simulink model "AdaptivePI_Simulation"  (R2020a)
settings: Solver=ode45  StartTime=0  StopTime=800  MaxStep=0.2  RelTol=1e-3  EnableMultiTasking=on
model workspace (MATLAB code in the model file):
  | %Model constants
  | k0                = 34930800;
  | DeltaER       = 5963.6;
  | DeltaH         = -11.92;
  | UA               = 0.3;
  | FV_plus_UA = 1.3;
  | 
  | %Fixed IC
  | Concentration0 = 1.5;
  | FeedCon0         = 10;
  | FeedTemp0       = 295;
  | 
  | %Derived IC
  | tmpVal = FeedCon0/Concentration0-1;
  | ReactorTemp0 = -DeltaER/log(tmpVal/k0);
  | CoolantTemp0 = (ReactorTemp0*(FV_plus_UA)+tmpVal*Concentration0*DeltaH-FeedTemp0)/UA;
  | 
  | %
  | tStep = 400; % [s] When the step reference change happens
  | Ts = 0.1; % [s] Sample time
  | 
  | % Scaling factors on the signals
  | CAscale = 10;
  | Tcscale = 1/10;
  | 
  | % Moving average filter
  | N = 100;
  | 
  | %Clean up
  | clear tmpVal
libraries: simulink x5
settings Model: OrderedModelArguments=off  Creator=The MathWorks, Inc.  LastModifiedBy=Mirza
settings DataIOCC: InitialState=[311.267; 8.5695]  SaveFormat=Array  SaveOutput=off  SignalLogging=off  DSMLogging=off  SaveTime=off  ReturnWorkspaceOutputs=off  SignalLoggingName=logsOut
settings OptimizationCC: BlockReduction=off  BooleanDataType=off  DefaultParameterBehavior=Inlined  InlineInvariantSignals=on  BufferReuse=off  ExpressionDepthLimit=2147483647  InitFltsAndDblsToZero=on  LifeSpan=inf
settings DebuggingCC: SaveWithParameterizedLinksMsg=none  UnderspecifiedInitializationDetection=Classic  MergeDetectMultiDrivingBlocksExec=none  CheckExecutionContextPreStartOutputMsg=on  CheckExecutionContextRuntimeOutputMsg=on  SignalResolutionControl=TryResolveAllWithWarning  MultiTaskDSMMsg=warning  MultiTaskCondExecSysMsg=none  FcnCallInpInsideContextMsg=warning  AllowSymbolicDim=off  StateNameClashWarn=warning  SFUnexpectedBacktrackingDiag=warning  SFNoUnconditionalDefaultTransitionDiag=warning  SFExecutionAtInitializationDiag=none  ArithmeticOperatorsInVariantConditions=warning
settings HardwareCC: ProdBitPerPointer=32  ProdBitPerSizeT=32  ProdBitPerPtrDiffT=32  ProdLargestAtomicFloat=None  ProdIntDivRoundTo=Undefined  ProdEndianess=Unspecified  ProdWordSize=32  ProdHWDeviceType=32-bit Generic  TargetUnknown=on
settings ModelReferenceCC: PropagateSignalLabelsOutOfModel=off
settings SFSimCC: SimUseLocalCustomCode=off  CustomCodeUndefinedFunction=UseInterfaceOnly
settings RTWCC: RTWUseLocalCustomCode=off
settings CodeAppCC: StateflowObjectComments=on
settings GRTTargetCC: TargetFcnLib=ansi_tfl_tmw.mat  TargetLangStandard=C89/C90 (ANSI)  CombineOutputUpdateFcns=off  GRTInterface=on
settings ConfigComp: CovMetricSettings=dw  CovHtmlReporting=on  CovSaveCumulativeToWorkspaceVar=on  CovSaveSingleToWorkspaceVar=on  CovExternalEMLEnable=off  CovSFcnEnable=off

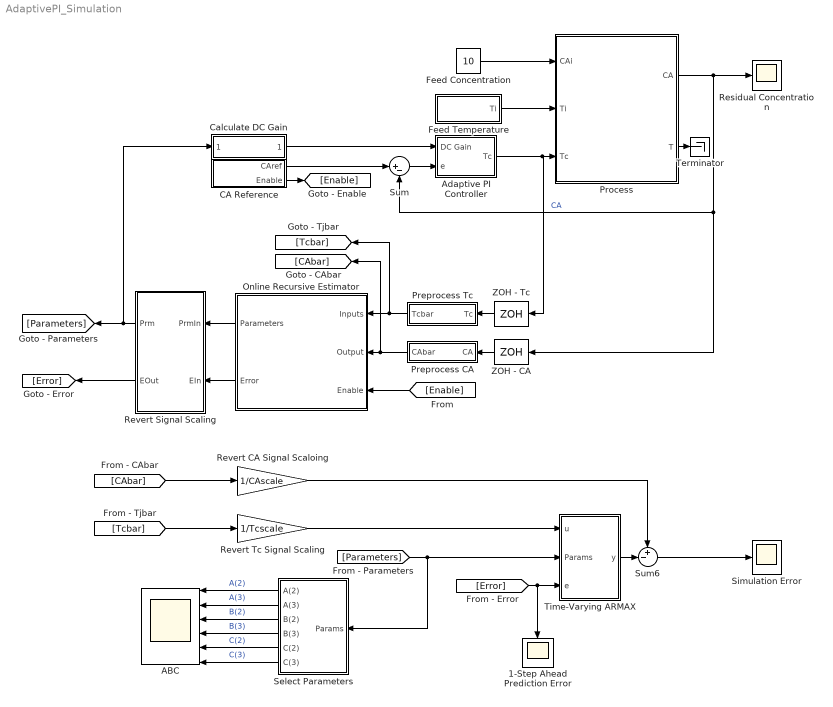
== system AdaptivePI_Simulation ==
  " Revert CA Signal Scaloing" : Gain  Gain=1/CAscale
  1-Step Ahead Prediction Error : Scope
  ABC : Scope  NumInputPorts=6
  Adaptive PI Controller : Subsystem
  CA Reference : Subsystem
  Calculate DC Gain : Subsystem
  Feed Concentration : Constant  Value=10
  Feed Temperature : Subsystem
  Online Recursive Estimator : Subsystem  mask{ModelStructure=ARMAX, A0=2, B0=[2], F0=2, C0=2, D0=2, d=[0], P0=100, History=Infinitna, WindowLength=2000, EstimationMethod=Faktor iscezavanja, Lambda=1 - 5e-3, ProcessNoiseCovariance=0.01, Tolerance=0.0001, AddEnablePort=on, EstimationError=on, ExcitationMeasure=off, SampleTime=0.1}
      mask prompts: ModelStructure "Izbor modela:"; A0 "Broj parametara u A(q) (na):"; B0 "Broj parametara u B(q) (nb):"; F0 "Broj parametara u F(q) (nf):"; C0 "Broj parametara u C(q) (nc):"; D0 "Broj parametara u D(q) (nd):"; d "Kasnjenje ulaza (nk):"; P0 "Matrica kovarijanse parametara:"; History "Historija:"; WindowLength "Sirina prozora:"; EstimationMethod "Metod estimacije:"; Lambda "Faktor iscezavanja:"; ProcessNoiseCovariance "Kovarijansa procesnog suma:"; Tolerance "Toleranca:"; AddEnablePort "Enable port"; EstimationError "Greska estimacije:"; ExcitationMeasure "Mjera pobude:"; SampleTime "Period uzorkovanja:"
      mask TypeOptions ModelStructure: ARX | ARMAX | BJ | OE
      mask Callback ModelStructure:
      | maskStr = get_param(gcb, 'ModelStructure');
      | maskStr1 = get_param(gcb, 'History');
      | maskStr2 = get_param(gcb, 'EstimationMethod');
      | 
      | if strcmp(maskStr, 'ARX') && strcmp(maskStr1, 'Infinitna') && strcmp(maskStr2, 'Faktor iscezavanja') ,
      |     set_param(gcb, 'MaskVisibilities', {'on';'on';'on';'off';'off';'off';'on';'on';'on';'off';'on';'on';'off';'off';'on';'on';'on';'on'}),
      | elseif strcmp(maskStr, 'ARX') && strcmp(maskStr1, 'Infinitna') && strcmp(maskStr2, 'BFGS') ,
      |     set_param(gcb, 'MaskVisibilities', {'on';'on';'on';'off';'off';'off';'on';'on';'on';'on';'on';'off';'off';'on';'on';'on';'on';'on'}),
      | elseif strcmp(maskStr, 'ARX') && strcmp(maskStr1, 'Infinitna') && strcmp(maskStr2, 'Kalmanov filter') ,
      |     set_param(gcb, 'MaskVisibilities', {'on';'on';'on';'off';'off';'off';'on';'on';'on';'off';'on';'off';'on';'off';'on';'on';'on';'on'}),
      | elseif strcmp(maskStr, 'ARX') && strcmp(maskStr1, 'Finitna') && strcmp(maskStr2, 'Faktor iscezavanja') ,
      |     set_param(gcb, 'MaskVisibilities', {'on';'on';'on';'off';'off';'off';'on';'on';'on';'on';'on';'off';'off';'off';'on';'on';'on';'on'}),
      | elseif strcmp(maskStr, 'ARX') && strcmp(maskStr1, 'Finitna') && strcmp(maskStr2, 'BFGS') ,
      |     set_param(gcb, 'MaskVisibilities', {'on';'on';'on';'off';'off';'off';'on';'on';'on';'on';'on';'off';'off';'on';'on';'on';'on';'on'}),
      | elseif strcmp(maskStr, 'ARX') && strcmp(maskStr1, 'Finitna') && strcmp(maskStr2, 'Kalmanov filter') ,
      |     set_param(gcb, 'MaskVisibilities', {'on';'on';'on';'off';'off';'off';'on';'on';'on';'on';'on';'off';'off';'off';'on';'on';'on';'on'}),
      | elseif strcmp(maskStr, 'ARMAX') && strcmp(maskStr1, 'Infinitna') && strcmp(maskStr2, 'Faktor iscezavanja') ,
      |     set_param(gcb, 'MaskVisibilities', {'on';'on';'on';'off';'on';'off';'on';'on';'on';'off';'on';'on';'off';'off';'on';'on';'on';'on'}),
      | elseif strcmp(maskStr, 'ARMAX') && strcmp(maskStr1, 'Infinitna') && strcmp(maskStr2, 'BFGS') ,
      |     set_param(gcb, 'MaskVisibilities', {'on';'on';'on';'off';'on';'off';'on';'on';'on';'on';'on';'off';'off';'on';'on';'on';'on';'on'}),
      | elseif strcmp(maskStr, 'ARMAX') && strcmp(maskStr1, 'Infinitna') && strcmp(maskStr2, 'Kalmanov filter') ,
      |     set_param(gcb, 'MaskVisibilities', {'on';'on';'on';'off';'on';'off';'on';'on';'on';'off';'on';'off';'on';'off';'on';'on';'on';'on'}),
      | elseif strcmp(maskStr, 'ARMAX') && strcmp(maskStr1, 'Finitna') && strcmp(maskStr2, 'Faktor iscezavanja') ,
      |     set_param(gcb, 'MaskVisibilities', {'on';'on';'on';'off';'on';'off';'on';'on';'on';'on';'on';'off';'off';'off';'on';'on';'on';'on'}),
      | elseif strcmp(maskStr, 'ARMAX') && strcmp(maskStr1, 'Finitna') && strcmp(maskStr2, 'BFGS') ,
      |     set_param(gcb, 'MaskVisibilities', {'on';'on';'on';'off';'on';'off';'on';'on';'on';'on';'on';'off';'off';'on';'on';'on';'on';'on'}),
      | elseif strcmp(maskStr, 'ARMAX') && strcmp(maskStr1, 'Finitna') && strcmp(maskStr2, 'Kalmanov filter') ,
      |     set_param(gcb, 'MaskVisibilities', {'on';'on';'on';'off';'on';'off';'on';'on';'on';'on';'on';'off';'off';'off';'on';'on';'on';'on'}),
      | elseif strcmp(maskStr, 'BJ') && strcmp(maskStr1, 'Infinitna') && strcmp(maskStr2, 'Faktor iscezavanja') ,
      |     set_param(gcb, 'MaskVisibilities', {'on';'off';'on';'on';'on';'on';'on';'on';'on';'off';'on';'on';'off';'off';'on';'on';'on';'on'}),
      | elseif strcmp(maskStr, 'BJ') && strcmp(maskStr1, 'Infinitna') && strcmp(maskStr2, 'BFGS') ,
      |     set_param(gcb, 'MaskVisibilities', {'on';'off';'on';'on';'on';'on';'on';'on';'on';'on';'on';'off';'off';'on';'on';'on';'on';'on'}),
      | elseif strcmp(maskStr, 'BJ') && strcmp(maskStr1, 'Infinitna') && strcmp(maskStr2, 'Kalmanov filter') ,
      |     set_param(gcb, 'MaskVisibilities', {'on';'off';'on';'on';'on';'on';'on';'on';'on';'off';'on';'off';'on';'off';'on';'on';'on';'on'}),
      | elseif strcmp(maskStr, 'BJ') && strcmp(maskStr1, 'Finitna') && strcmp(maskStr2, 'Faktor iscezavanja') ,
      |     set_param(gcb, 'MaskVisibilities', {'on';'off';'on';'on';'on';'on';'on';'on';'on';'on';'on';'off';'off';'off';'on';'on';'on';'on'}),
      | elseif strcmp(maskStr, 'BJ') && strcmp(maskStr1, 'Finitna') && strcmp(maskStr2, 'BFGS') ,
      |     set_param(gcb, 'MaskVisibilities', {'on';'off';'on';'on';'on';'on';'on';'on';'on';'on';'on';'off';'off';'on';'on';'on';'on';'on'}),
      | elseif strcmp(maskStr, 'BJ') && strcmp(maskStr1, 'Finitna') && strcmp(maskStr2, 'Kalmanov filter') ,
      |     set_param(gcb, 'MaskVisibilities', {'on';'off';'on';'on';'on';'on';'on';'on';'on';'on';'on';'off';'off';'off';'on';'on';'on';'on'}),
      | elseif strcmp(maskStr, 'OE') && strcmp(maskStr1, 'Infinitna') && strcmp(maskStr2, 'Faktor iscezavanja') ,
      |     set_param(gcb, 'MaskVisibilities', {'on';'off';'on';'on';'off';'off';'on';'on';'on';'off';'on';'on';'off';'off';'on';'on';'on';'on'}),
      | elseif strcmp(maskStr, 'OE') && strcmp(maskStr1, 'Infinitna') && strcmp(maskStr2, 'BFGS') ,
      |     set_param(gcb, 'MaskVisibilities', {'on';'off';'on';'on';'off';'off';'on';'on';'on';'on';'on';'off';'off';'on';'on';'on';'on';'on'}),
      | elseif strcmp(maskStr, 'OE') && strcmp(maskStr1, 'Infinitna') && strcmp(maskStr2, 'Kalmanov filter') ,
      |     set_param(gcb, 'MaskVisibilities', {'on';'off';'on';'on';'off';'off';'on';'on';'on';'off';'on';'off';'on';'off';'on';'on';'on';'on'}),
      | elseif strcmp(maskStr, 'OE') && strcmp(maskStr1, 'Finitna') && strcmp(maskStr2, 'Faktor iscezavanja') ,
      |     set_param(gcb, 'MaskVisibilities', {'on';'off';'on';'on';'off';'off';'on';'on';'on';'on';'on';'off';'off';'off';'on';'on';'on';'on'}),
      | elseif strcmp(maskStr, 'OE') && strcmp(maskStr1, 'Finitna') && strcmp(maskStr2, 'BFGS') ,
      |     set_param(gcb, 'MaskVisibilities', {'on';'off';'on';'on';'off';'off';'on';'on';'on';'on';'on';'off';'off';'on';'on';'on';'on';'on'}),
      | elseif strcmp(maskStr, 'OE') && strcmp(maskStr1, 'Finitna') && strcmp(maskStr2, 'Kalmanov filter') ,
      |     set_param(gcb, 'MaskVisibilities', {'on';'off';'on';'on';'off';'off';'on';'on';'on';'on';'on';'off';'off';'off';'on';'on';'on';'on'}),
      | end
      mask TypeOptions History: Infinitna | Finitna
      mask Callback History:
      | maskStr = get_param(gcb, 'ModelStructure');
      | maskStr1 = get_param(gcb, 'History');
      | maskStr2 = get_param(gcb, 'EstimationMethod');
      | 
      | if strcmp(maskStr, 'ARX') && strcmp(maskStr1, 'Infinitna') && strcmp(maskStr2, 'Faktor iscezavanja') ,
      |     set_param(gcb, 'MaskVisibilities', {'on';'on';'on';'off';'off';'off';'on';'on';'on';'off';'on';'on';'off';'off';'on';'on';'on';'on'}),
      | elseif strcmp(maskStr, 'ARX') && strcmp(maskStr1, 'Infinitna') && strcmp(maskStr2, 'BFGS') ,
      |     set_param(gcb, 'MaskVisibilities', {'on';'on';'on';'off';'off';'off';'on';'on';'on';'on';'on';'off';'off';'on';'on';'on';'on';'on'}),
      | elseif strcmp(maskStr, 'ARX') && strcmp(maskStr1, 'Infinitna') && strcmp(maskStr2, 'Kalmanov filter') ,
      |     set_param(gcb, 'MaskVisibilities', {'on';'on';'on';'off';'off';'off';'on';'on';'on';'off';'on';'off';'on';'off';'on';'on';'on';'on'}),
      | elseif strcmp(maskStr, 'ARX') && strcmp(maskStr1, 'Finitna') && strcmp(maskStr2, 'Faktor iscezavanja') ,
      |     set_param(gcb, 'MaskVisibilities', {'on';'on';'on';'off';'off';'off';'on';'on';'on';'on';'on';'off';'off';'off';'on';'on';'on';'on'}),
      | elseif strcmp(maskStr, 'ARX') && strcmp(maskStr1, 'Finitna') && strcmp(maskStr2, 'BFGS') ,
      |     set_param(gcb, 'MaskVisibilities', {'on';'on';'on';'off';'off';'off';'on';'on';'on';'on';'on';'off';'off';'on';'on';'on';'on';'on'}),
      | elseif strcmp(maskStr, 'ARX') && strcmp(maskStr1, 'Finitna') && strcmp(maskStr2, 'Kalmanov filter') ,
      |     set_param(gcb, 'MaskVisibilities', {'on';'on';'on';'off';'off';'off';'on';'on';'on';'on';'on';'off';'off';'off';'on';'on';'on';'on'}),
      | elseif strcmp(maskStr, 'ARMAX') && strcmp(maskStr1, 'Infinitna') && strcmp(maskStr2, 'Faktor iscezavanja') ,
      |     set_param(gcb, 'MaskVisibilities', {'on';'on';'on';'off';'on';'off';'on';'on';'on';'off';'on';'on';'off';'off';'on';'on';'on';'on'}),
      | elseif strcmp(maskStr, 'ARMAX') && strcmp(maskStr1, 'Infinitna') && strcmp(maskStr2, 'BFGS') ,
      |     set_param(gcb, 'MaskVisibilities', {'on';'on';'on';'off';'on';'off';'on';'on';'on';'on';'on';'off';'off';'on';'on';'on';'on';'on'}),
      | elseif strcmp(maskStr, 'ARMAX') && strcmp(maskStr1, 'Infinitna') && strcmp(maskStr2, 'Kalmanov filter') ,
      |     set_param(gcb, 'MaskVisibilities', {'on';'on';'on';'off';'on';'off';'on';'on';'on';'off';'on';'off';'on';'off';'on';'on';'on';'on'}),
      | elseif strcmp(maskStr, 'ARMAX') && strcmp(maskStr1, 'Finitna') && strcmp(maskStr2, 'Faktor iscezavanja') ,
      |     set_param(gcb, 'MaskVisibilities', {'on';'on';'on';'off';'on';'off';'on';'on';'on';'on';'on';'off';'off';'off';'on';'on';'on';'on'}),
      | elseif strcmp(maskStr, 'ARMAX') && strcmp(maskStr1, 'Finitna') && strcmp(maskStr2, 'BFGS') ,
      |     set_param(gcb, 'MaskVisibilities', {'on';'on';'on';'off';'on';'off';'on';'on';'on';'on';'on';'off';'off';'on';'on';'on';'on';'on'}),
      | elseif strcmp(maskStr, 'ARMAX') && strcmp(maskStr1, 'Finitna') && strcmp(maskStr2, 'Kalmanov filter') ,
      |     set_param(gcb, 'MaskVisibilities', {'on';'on';'on';'off';'on';'off';'on';'on';'on';'on';'on';'off';'off';'off';'on';'on';'on';'on'}),
      | elseif strcmp(maskStr, 'BJ') && strcmp(maskStr1, 'Infinitna') && strcmp(maskStr2, 'Faktor iscezavanja') ,
      |     set_param(gcb, 'MaskVisibilities', {'on';'off';'on';'on';'on';'on';'on';'on';'on';'off';'on';'on';'off';'off';'on';'on';'on';'on'}),
      | elseif strcmp(maskStr, 'BJ') && strcmp(maskStr1, 'Infinitna') && strcmp(maskStr2, 'BFGS') ,
      |     set_param(gcb, 'MaskVisibilities', {'on';'off';'on';'on';'on';'on';'on';'on';'on';'on';'on';'off';'off';'on';'on';'on';'on';'on'}),
      | elseif strcmp(maskStr, 'BJ') && strcmp(maskStr1, 'Infinitna') && strcmp(maskStr2, 'Kalmanov filter') ,
      |     set_param(gcb, 'MaskVisibilities', {'on';'off';'on';'on';'on';'on';'on';'on';'on';'off';'on';'off';'on';'off';'on';'on';'on';'on'}),
      | elseif strcmp(maskStr, 'BJ') && strcmp(maskStr1, 'Finitna') && strcmp(maskStr2, 'Faktor iscezavanja') ,
      |     set_param(gcb, 'MaskVisibilities', {'on';'off';'on';'on';'on';'on';'on';'on';'on';'on';'on';'off';'off';'off';'on';'on';'on';'on'}),
      | elseif strcmp(maskStr, 'BJ') && strcmp(maskStr1, 'Finitna') && strcmp(maskStr2, 'BFGS') ,
      |     set_param(gcb, 'MaskVisibilities', {'on';'off';'on';'on';'on';'on';'on';'on';'on';'on';'on';'off';'off';'on';'on';'on';'on';'on'}),
      | elseif strcmp(maskStr, 'BJ') && strcmp(maskStr1, 'Finitna') && strcmp(maskStr2, 'Kalmanov filter') ,
      |     set_param(gcb, 'MaskVisibilities', {'on';'off';'on';'on';'on';'on';'on';'on';'on';'on';'on';'off';'off';'off';'on';'on';'on';'on'}),
      | elseif strcmp(maskStr, 'OE') && strcmp(maskStr1, 'Infinitna') && strcmp(maskStr2, 'Faktor iscezavanja') ,
      |     set_param(gcb, 'MaskVisibilities', {'on';'off';'on';'on';'off';'off';'on';'on';'on';'off';'on';'on';'off';'off';'on';'on';'on';'on'}),
      | elseif strcmp(maskStr, 'OE') && strcmp(maskStr1, 'Infinitna') && strcmp(maskStr2, 'BFGS') ,
      |     set_param(gcb, 'MaskVisibilities', {'on';'off';'on';'on';'off';'off';'on';'on';'on';'on';'on';'off';'off';'on';'on';'on';'on';'on'}),
      | elseif strcmp(maskStr, 'OE') && strcmp(maskStr1, 'Infinitna') && strcmp(maskStr2, 'Kalmanov filter') ,
      |     set_param(gcb, 'MaskVisibilities', {'on';'off';'on';'on';'off';'off';'on';'on';'on';'off';'on';'off';'on';'off';'on';'on';'on';'on'}),
      | elseif strcmp(maskStr, 'OE') && strcmp(maskStr1, 'Finitna') && strcmp(maskStr2, 'Faktor iscezavanja') ,
      |     set_param(gcb, 'MaskVisibilities', {'on';'off';'on';'on';'off';'off';'on';'on';'on';'on';'on';'off';'off';'off';'on';'on';'on';'on'}),
      | elseif strcmp(maskStr, 'OE') && strcmp(maskStr1, 'Finitna') && strcmp(maskStr2, 'BFGS') ,
      |     set_param(gcb, 'MaskVisibilities', {'on';'off';'on';'on';'off';'off';'on';'on';'on';'on';'on';'off';'off';'on';'on';'on';'on';'on'}),
      | elseif strcmp(maskStr, 'OE') && strcmp(maskStr1, 'Finitna') && strcmp(maskStr2, 'Kalmanov filter') ,
      |     set_param(gcb, 'MaskVisibilities', {'on';'off';'on';'on';'off';'off';'on';'on';'on';'on';'on';'off';'off';'off';'on';'on';'on';'on'}),
      | end
      mask TypeOptions EstimationMethod: Faktor iscezavanja | BFGS | Kalmanov filter
      mask Callback EstimationMethod:
      | maskStr = get_param(gcb, 'ModelStructure');
      | maskStr1 = get_param(gcb, 'History');
      | maskStr2 = get_param(gcb, 'EstimationMethod');
      | 
      | if strcmp(maskStr, 'ARX') && strcmp(maskStr1, 'Infinitna') && strcmp(maskStr2, 'Faktor iscezavanja') ,
      |     set_param(gcb, 'MaskVisibilities', {'on';'on';'on';'off';'off';'off';'on';'on';'on';'off';'on';'on';'off';'off';'on';'on';'on';'on'}),
      | elseif strcmp(maskStr, 'ARX') && strcmp(maskStr1, 'Infinitna') && strcmp(maskStr2, 'BFGS') ,
      |     set_param(gcb, 'MaskVisibilities', {'on';'on';'on';'off';'off';'off';'on';'on';'on';'on';'on';'off';'off';'on';'on';'on';'on';'on'}),
      | elseif strcmp(maskStr, 'ARX') && strcmp(maskStr1, 'Infinitna') && strcmp(maskStr2, 'Kalmanov filter') ,
      |     set_param(gcb, 'MaskVisibilities', {'on';'on';'on';'off';'off';'off';'on';'on';'on';'off';'on';'off';'on';'off';'on';'on';'on';'on'}),
      | elseif strcmp(maskStr, 'ARX') && strcmp(maskStr1, 'Finitna') && strcmp(maskStr2, 'Faktor iscezavanja') ,
      |     set_param(gcb, 'MaskVisibilities', {'on';'on';'on';'off';'off';'off';'on';'on';'on';'on';'on';'off';'off';'off';'on';'on';'on';'on'}),
      | elseif strcmp(maskStr, 'ARX') && strcmp(maskStr1, 'Finitna') && strcmp(maskStr2, 'BFGS') ,
      |     set_param(gcb, 'MaskVisibilities', {'on';'on';'on';'off';'off';'off';'on';'on';'on';'on';'on';'off';'off';'on';'on';'on';'on';'on'}),
      | elseif strcmp(maskStr, 'ARX') && strcmp(maskStr1, 'Finitna') && strcmp(maskStr2, 'Kalmanov filter') ,
      |     set_param(gcb, 'MaskVisibilities', {'on';'on';'on';'off';'off';'off';'on';'on';'on';'on';'on';'off';'off';'off';'on';'on';'on';'on'}),
      | elseif strcmp(maskStr, 'ARMAX') && strcmp(maskStr1, 'Infinitna') && strcmp(maskStr2, 'Faktor iscezavanja') ,
      |     set_param(gcb, 'MaskVisibilities', {'on';'on';'on';'off';'on';'off';'on';'on';'on';'off';'on';'on';'off';'off';'on';'on';'on';'on'}),
      | elseif strcmp(maskStr, 'ARMAX') && strcmp(maskStr1, 'Infinitna') && strcmp(maskStr2, 'BFGS') ,
      |     set_param(gcb, 'MaskVisibilities', {'on';'on';'on';'off';'on';'off';'on';'on';'on';'on';'on';'off';'off';'on';'on';'on';'on';'on'}),
      | elseif strcmp(maskStr, 'ARMAX') && strcmp(maskStr1, 'Infinitna') && strcmp(maskStr2, 'Kalmanov filter') ,
      |     set_param(gcb, 'MaskVisibilities', {'on';'on';'on';'off';'on';'off';'on';'on';'on';'off';'on';'off';'on';'off';'on';'on';'on';'on'}),
      | elseif strcmp(maskStr, 'ARMAX') && strcmp(maskStr1, 'Finitna') && strcmp(maskStr2, 'Faktor iscezavanja') ,
      |     set_param(gcb, 'MaskVisibilities', {'on';'on';'on';'off';'on';'off';'on';'on';'on';'on';'on';'off';'off';'off';'on';'on';'on';'on'}),
      | elseif strcmp(maskStr, 'ARMAX') && strcmp(maskStr1, 'Finitna') && strcmp(maskStr2, 'BFGS') ,
      |     set_param(gcb, 'MaskVisibilities', {'on';'on';'on';'off';'on';'off';'on';'on';'on';'on';'on';'off';'off';'on';'on';'on';'on';'on'}),
      | elseif strcmp(maskStr, 'ARMAX') && strcmp(maskStr1, 'Finitna') && strcmp(maskStr2, 'Kalmanov filter') ,
      |     set_param(gcb, 'MaskVisibilities', {'on';'on';'on';'off';'on';'off';'on';'on';'on';'on';'on';'off';'off';'off';'on';'on';'on';'on'}),
      | elseif strcmp(maskStr, 'BJ') && strcmp(maskStr1, 'Infinitna') && strcmp(maskStr2, 'Faktor iscezavanja') ,
      |     set_param(gcb, 'MaskVisibilities', {'on';'off';'on';'on';'on';'on';'on';'on';'on';'off';'on';'on';'off';'off';'on';'on';'on';'on'}),
      | elseif strcmp(maskStr, 'BJ') && strcmp(maskStr1, 'Infinitna') && strcmp(maskStr2, 'BFGS') ,
      |     set_param(gcb, 'MaskVisibilities', {'on';'off';'on';'on';'on';'on';'on';'on';'on';'on';'on';'off';'off';'on';'on';'on';'on';'on'}),
      | elseif strcmp(maskStr, 'BJ') && strcmp(maskStr1, 'Infinitna') && strcmp(maskStr2, 'Kalmanov filter') ,
      |     set_param(gcb, 'MaskVisibilities', {'on';'off';'on';'on';'on';'on';'on';'on';'on';'off';'on';'off';'on';'off';'on';'on';'on';'on'}),
      | elseif strcmp(maskStr, 'BJ') && strcmp(maskStr1, 'Finitna') && strcmp(maskStr2, 'Faktor iscezavanja') ,
      |     set_param(gcb, 'MaskVisibilities', {'on';'off';'on';'on';'on';'on';'on';'on';'on';'on';'on';'off';'off';'off';'on';'on';'on';'on'}),
      | elseif strcmp(maskStr, 'BJ') && strcmp(maskStr1, 'Finitna') && strcmp(maskStr2, 'BFGS') ,
      |     set_param(gcb, 'MaskVisibilities', {'on';'off';'on';'on';'on';'on';'on';'on';'on';'on';'on';'off';'off';'on';'on';'on';'on';'on'}),
      | elseif strcmp(maskStr, 'BJ') && strcmp(maskStr1, 'Finitna') && strcmp(maskStr2, 'Kalmanov filter') ,
      |     set_param(gcb, 'MaskVisibilities', {'on';'off';'on';'on';'on';'on';'on';'on';'on';'on';'on';'off';'off';'off';'on';'on';'on';'on'}),
      | elseif strcmp(maskStr, 'OE') && strcmp(maskStr1, 'Infinitna') && strcmp(maskStr2, 'Faktor iscezavanja') ,
      |     set_param(gcb, 'MaskVisibilities', {'on';'off';'on';'on';'off';'off';'on';'on';'on';'off';'on';'on';'off';'off';'on';'on';'on';'on'}),
      | elseif strcmp(maskStr, 'OE') && strcmp(maskStr1, 'Infinitna') && strcmp(maskStr2, 'BFGS') ,
      |     set_param(gcb, 'MaskVisibilities', {'on';'off';'on';'on';'off';'off';'on';'on';'on';'on';'on';'off';'off';'on';'on';'on';'on';'on'}),
      | elseif strcmp(maskStr, 'OE') && strcmp(maskStr1, 'Infinitna') && strcmp(maskStr2, 'Kalmanov filter') ,
      |     set_param(gcb, 'MaskVisibilities', {'on';'off';'on';'on';'off';'off';'on';'on';'on';'off';'on';'off';'on';'off';'on';'on';'on';'on'}),
      | elseif strcmp(maskStr, 'OE') && strcmp(maskStr1, 'Finitna') && strcmp(maskStr2, 'Faktor iscezavanja') ,
      |     set_param(gcb, 'MaskVisibilities', {'on';'off';'on';'on';'off';'off';'on';'on';'on';'on';'on';'off';'off';'off';'on';'on';'on';'on'}),
      | elseif strcmp(maskStr, 'OE') && strcmp(maskStr1, 'Finitna') && strcmp(maskStr2, 'BFGS') ,
      |     set_param(gcb, 'MaskVisibilities', {'on';'off';'on';'on';'off';'off';'on';'on';'on';'on';'on';'off';'off';'on';'on';'on';'on';'on'}),
      | elseif strcmp(maskStr, 'OE') && strcmp(maskStr1, 'Finitna') && strcmp(maskStr2, 'Kalmanov filter') ,
      |     set_param(gcb, 'MaskVisibilities', {'on';'off';'on';'on';'off';'off';'on';'on';'on';'on';'on';'off';'off';'off';'on';'on';'on';'on'}),
      | end
      mask Callback AddEnablePort:
      | maskStr3 = get_param(gcb, 'AddEnablePort');
      | 
      | if strcmp(maskStr3, 'on')
      |      if (getSimulinkBlockHandle('PSAU_SeminarskiRad_AdaptivePI/Online Recursive Estimator/EnableConst')>0)
      |           delete_line('PSAU_SeminarskiRad_AdaptivePI/Online Recursive Estimator', 'EnableConst/1', 'Data Type Conversion/1');
      |           delete_block('PSAU_SeminarskiRad_AdaptivePI/Online Recursive Estimator/EnableConst');
      |      end
      |      if (getSimulinkBlockHandle('PSAU_SeminarskiRad_AdaptivePI/Online Recursive Estimator/Enable')==-1)
      |           add_block('simulink/Sources/In1','PSAU_SeminarskiRad_AdaptivePI/Online Recursive Estimator/Enable');
      |           set_param('PSAU_SeminarskiRad_AdaptivePI/Online Recursive Estimator/Enable','position',[510, 403, 540, 417]);
      |           add_line('PSAU_SeminarskiRad_AdaptivePI/Online Recursive Estimator', 'Enable/1', 'Data Type Conversion/1');
      |      end
      | elseif strcmp(maskStr3, 'off')
      |     if (getSimulinkBlockHandle('PSAU_SeminarskiRad_AdaptivePI/Online Recursive Estimator/Enable')>0)
      |          delete_line('PSAU_SeminarskiRad_AdaptivePI/Online Recursive Estimator', 'Enable/1', 'Data Type Conversion/1');
      |          delete_block('PSAU_SeminarskiRad_AdaptivePI/Online Recursive Estimator/Enable');
      |     end
      |     if (getSimulinkBlockHandle('PSAU_SeminarskiRad_AdaptivePI/Online Recursive Estimator/EnableConst')==-1)
      |          add_block('simulink/Sources/Constant','PSAU_SeminarskiRad_AdaptivePI/Online Recursive Estimator/EnableConst');
      |          set_param('PSAU_SeminarskiRad_AdaptivePI/Online Recursive Estimator/EnableConst','position',[510, 395, 540, 425]);
      |          add_line('PSAU_SeminarskiRad_AdaptivePI/Online Recursive Estimator', 'EnableConst/1', 'Data Type Conversion/1');
      |     end
      | end
      mask Callback EstimationError:
      | maskStr4 = get_param(gcb, 'EstimationError');
      | 
      | if strcmp(maskStr4, 'on')
      |      if (getSimulinkBlockHandle('PSAU_SeminarskiRad_AdaptivePI/Online Recursive Estimator/ETerminator')>0)
      |           delete_line('PSAU_SeminarskiRad_AdaptivePI/Online Recursive Estimator', 'sf/2', 'ETerminator/1');
      |           delete_block('PSAU_SeminarskiRad_AdaptivePI/Online Recursive Estimator/ETerminator');
      |      end
      |      if (getSimulinkBlockHandle('PSAU_SeminarskiRad_AdaptivePI/Online Recursive Estimator/Error')==-1)
      |           add_block('simulink/Sinks/Out1','PSAU_SeminarskiRad_AdaptivePI/Online Recursive Estimator/Error');
      |           set_param('PSAU_SeminarskiRad_AdaptivePI/Online Recursive Estimator/Error','position',[1080, 335, 1110, 365]);
      |           add_line('PSAU_SeminarskiRad_AdaptivePI/Online Recursive Estimator', 'sf/2', 'Error/1');
      |      end
      | elseif strcmp(maskStr4, 'off')
      |     if (getSimulinkBlockHandle('PSAU_SeminarskiRad_AdaptivePI/Online Recursive Estimator/Error')>0)
      |          delete_line('PSAU_SeminarskiRad_AdaptivePI/Online Recursive Estimator', 'sf/2', 'Error/1');
      |          delete_block('PSAU_SeminarskiRad_AdaptivePI/Online Recursive Estimator/Error');
      |     end
      |     if (getSimulinkBlockHandle('PSAU_SeminarskiRad_AdaptivePI/Online Recursive Estimator/ETerminator')==-1)
      |          add_block('simulink/Commonly Used Blocks/Terminator','PSAU_SeminarskiRad_AdaptivePI/Online Recursive Estimator/ETerminator');
      |          set_param('PSAU_SeminarskiRad_AdaptivePI/Online Recursive Estimator/ETerminator','position',[1080, 335, 1110, 365]);
      |          add_line('PSAU_SeminarskiRad_AdaptivePI/Online Recursive Estimator', 'sf/2', 'ETerminator/1');
      |     end
      | end
      mask Callback ExcitationMeasure:
      | maskStr5 = get_param(gcb, 'ExcitationMeasure');
      | 
      | if strcmp(maskStr5, 'on')
      |      if (getSimulinkBlockHandle('PSAU_SeminarskiRad_AdaptivePI/Online Recursive Estimator/ExTerminator')>0)
      |           delete_line('PSAU_SeminarskiRad_AdaptivePI/Online Recursive Estimator', 'sf/3', 'ExTerminator/1');
      |           delete_block('PSAU_SeminarskiRad_AdaptivePI/Online Recursive Estimator/ExTerminator');
      |      end
      |      if (getSimulinkBlockHandle('PSAU_SeminarskiRad_AdaptivePI/Online Recursive Estimator/Excitation')==-1)
      |           add_block('simulink/Sinks/Out1','PSAU_SeminarskiRad_AdaptivePI/Online Recursive Estimator/Excitation');
      |           set_param('PSAU_SeminarskiRad_AdaptivePI/Online Recursive Estimator/Excitation','position',[1080, 403, 1110, 417]);
      |           add_line('PSAU_SeminarskiRad_AdaptivePI/Online Recursive Estimator', 'sf/3', 'Excitation/1');
      |      end
      | elseif strcmp(maskStr5, 'off')
      |     if (getSimulinkBlockHandle('PSAU_SeminarskiRad_AdaptivePI/Online Recursive Estimator/Excitation')>0)
      |          delete_line('PSAU_SeminarskiRad_AdaptivePI/Online Recursive Estimator', 'sf/3', 'Excitation/1');
      |          delete_block('PSAU_SeminarskiRad_AdaptivePI/Online Recursive Estimator/Excitation');
      |     end
      |     if (getSimulinkBlockHandle('PSAU_SeminarskiRad_AdaptivePI/Online Recursive Estimator/ExTerminator')==-1)
      |          add_block('simulink/Commonly Used Blocks/Terminator','PSAU_SeminarskiRad_AdaptivePI/Online Recursive Estimator/ExTerminator');
      |          set_param('PSAU_SeminarskiRad_AdaptivePI/Online Recursive Estimator/ExTerminator','position',[1080, 403, 1110, 417]);
      |          add_line('PSAU_SeminarskiRad_AdaptivePI/Online Recursive Estimator', 'sf/3', 'ExTerminator/1');
      |     end
      | end
      mask DialogControl DescGroupVar Prompt: Rekurzivna estimacija parametara
      mask DialogControl DescTextVar Prompt: Blok za estimaciju parametara linearnih modela sa ARX, ARMAX, BJ i OE strukturom.
      mask DialogControl ContainerModelParameters Prompt: Parametri modela
      mask DialogControl ContainerModelStructure Prompt: Opis modela
      mask DialogControl ContainerAlgorithmAndBlockOptions Prompt: Opcije bloka i algoritma
      mask DialogControl ContainerAlgorithmOptions Prompt: Opcije algoritma
  Preprocess CA : Subsystem
  Preprocess Tc : Subsystem
  Process : Subsystem
  Residual Concentration : Scope
  Revert Signal Scaling : Subsystem
  Revert Tc Signal Scaling : Gain  Gain=1/Tcscale
  Select Parameters : Subsystem
  Simulation Error : Scope
  Sum : Sum  Inputs=|+-
  Sum6 : Sum  Inputs=+-|
  Terminator : Terminator
  Time-Varying ARMAX : Subsystem
  ZOH - CA : ZeroOrderHold  SampleTime=Ts
  ZOH - Tc : ZeroOrderHold  SampleTime=Ts
  wires:
  Process/2(T) -> Terminator/1
  Preprocess Tc/1(Tcbar) -> Online Recursive Estimator/1(Inputs), [Tcbar]
  Preprocess CA/1(CAbar) -> [CAbar], Online Recursive Estimator/2(Output)
  Process/1(CA) -> Residual Concentration/1, ZOH - CA/1, Sum/2  "CA"
  Feed Concentration/1 -> Process/1(CAi)
  CA Reference/1(CAref) -> Sum/1
  Feed Temperature/1(Ti) -> Process/2(Ti)
  CA Reference/2(Enable) -> [Enable]
  Revert Signal Scaling/1(Prm) -> [Parameters], Calculate DC Gain/1(Params)
  ZOH - Tc/1 -> Preprocess Tc/1(Tc)
  ZOH - CA/1 -> Preprocess CA/1(CA)
  Adaptive PI Controller/1(Tc) -> ZOH - Tc/1, Process/3(Tc)
  Calculate DC Gain/1(DCGain) -> Adaptive PI Controller/1(DC Gain)
  Sum/1 -> Adaptive PI Controller/2(e)
  Revert Signal Scaling/2(EOut) -> [Error]
  [Parameters] -> Select Parameters/1(Params), Time-Varying ARMAX/2(Params)
  [Error] -> Time-Varying ARMAX/3(e), 1-Step Ahead Prediction Error/1
  Revert Tc Signal Scaling/1 -> Time-Varying ARMAX/1(u)
  [Tcbar] -> Revert Tc Signal Scaling/1
  [CAbar] -> " Revert CA Signal Scaloing"/1
  " Revert CA Signal Scaloing"/1 -> Sum6/1
  Time-Varying ARMAX/1(y) -> Sum6/2
  Select Parameters/4(B(3)) -> ABC/4  "B(3)"
  Select Parameters/3(B(2)) -> ABC/3  "B(2)"
  Select Parameters/5(C(2)) -> ABC/5  "C(2)"
  Select Parameters/2(A(3)) -> ABC/2  "A(3)"
  Select Parameters/6(C(3)) -> ABC/6  "C(3)"
  Select Parameters/1(A(2)) -> ABC/1  "A(2)"
  Sum6/1 -> Simulation Error/1
  Online Recursive Estimator/1(Parameters) -> Revert Signal Scaling/1(PrmIn)
  [Enable] -> Online Recursive Estimator/3(Enable)
  Online Recursive Estimator/2(Error) -> Revert Signal Scaling/2(EIn)

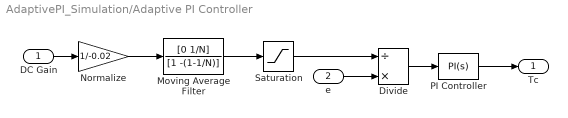
== system AdaptivePI_Simulation/Adaptive PI Controller ==
  DC Gain : Inport
  e : Inport  Port=2
  Divide : Product  Inputs=/*
  Moving Average Filter : DiscreteFilter  Numerator=[0 1/N]  Denominator=[1 -(1-1/N)]  InitialStates=N  SampleTime=Ts
  Normalize : Gain  Gain=1/-0.02
  PI Controller : simulink/Continuous/PID Controller  Controller=PI  Form=Parallel  TimeDomain=Continuous-time  UseExternalTs=off  SampleTime=-1  IntegratorMethod=Forward Euler  FilterMethod=Forward Euler  ControllerParametersSource=internal  P=-13  I=-25  D=0  UseFilter=on  N=100  TunerSelectOption=Transfer Function Based (PID Tuner App)  InitialConditionSource=internal  InitialConditionForIntegrator=CoolantTemp0  InitialConditionForFilter=0  DifferentiatorICPrevScaledInput=0  ExternalReset=none  TrackingMode=off  Kt=1  LimitOutput=off  UpperSaturationLimit=inf  LowerSaturationLimit=-inf  LinearizeAsGain=on  AntiWindupMode=none  Kb=1  POutMin=[]  POutMax=[]  IOutMin=[]  IOutMax=[]  DOutMin=[]  DOutMax=[]  NOutMin=[]  NOutMax=[]  SumOutMin=[]  SumOutMax=[]  SaturationOutMin=[]  SaturationOutMax=[]  PParamMin=[]  PParamMax=[]  IParamMin=[]  IParamMax=[]  DParamMin=[]  DParamMax=[]  NParamMin=[]  NParamMax=[]  KbParamMin=[]  KbParamMax=[]  KtParamMin=[]  KtParamMax=[]  KbOutMin=[]  KbOutMax=[]  KtOutMin=[]  KtOutMax=[]  IntegratorOutMin=[]  IntegratorOutMax=[]  FilterOutMin=[]  FilterOutMax=[]  SumI1OutMin=[]  SumI1OutMax=[]  SumI2OutMin=[]  SumI2OutMax=[]  SumI3OutMin=[]  SumI3OutMax=[]  SumI4OutMin=[]  SumI4OutMax=[]  SumDOutMin=[]  SumDOutMax=[]  DifferentiatorOutMin=[]  DifferentiatorOutMax=[]  FilterDiffOutCoefMin=[]  FilterDiffOutCoefMax=[]  ReciprocalOutMin=[]  ReciprocalOutMax=[]  SumDenOutMin=[]  SumDenOutMax=[]  SumNumOutMin=[]  SumNumOutMax=[]  DivideOutMin=[]  DivideOutMax=[]  UdiffTsProdOutMin=[]  UdiffTsProdOutMax=[]  NTsProdOutMin=[]  NTsProdOutMax=[]  UintegralTsProdOutMin=[]  UintegralTsProdOutMax=[]  UngainTsProdOutMin=[]  UngainTsProdOutMax=[]  IntegratorContinuousStateAttributes=''  IntegratorStateMustResolveToSignalObject=off  IntegratorRTWStateStorageClass=Auto  FilterContinuousStateAttributes=''  FilterStateMustResolveToSignalObject=off  FilterRTWStateStorageClass=Auto  ParallelPVariant=InternalParameters  IdealPVariant=Disabled  IVariant=InternalParameters  DVariant=Disabled  IntegratorVariant=Continuous  SatVariant=Disabled  AWVariant=Passthrough  PCopyVariant=Disabled  TRVariant=Disabled  FdbkBlocksVariant=Forward  IdealPFdbkVariant=Disabled  SatFdbkVariant=Disabled  DerivativeFilterVariant=Disabled  NVariant=Disabled  NCopyVariant=Disabled_SignalSpec  FilterICVariant=Disabled  IntegratorICVariant=InternalICs  ExternalResetVariant=Disabled  TRSumVariant=Passthrough  SumFdbkVariant=Disabled  SumVariant=Sum_PI  TsampFilterVariant=InternalTs  TsampNgainVariant=Passthrough  TsampIntegralVariant=Passthrough
  Saturation : Saturate  UpperLimit=3  LowerLimit=0.5
  Tc : Outport  VectorParamsAs1DForOutWhenUnconnected=off
  wires:
  e/1 -> Divide/2
  Divide/1 -> PI Controller/1
  PI Controller/1 -> Tc/1
  Moving Average Filter/1 -> Saturation/1
  DC Gain/1 -> Normalize/1
  Normalize/1 -> Moving Average Filter/1
  Saturation/1 -> Divide/1

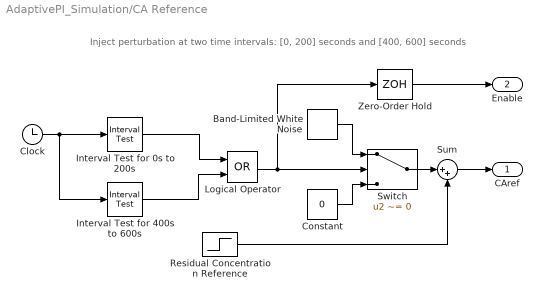
== system AdaptivePI_Simulation/CA Reference ==
  note: Inject perturbation at two time intervals: [0, 200] seconds and [400, 600] seconds
  Band-Limited White Noise : simulink/Sources/Band-Limited White Noise  Cov=0.015  Ts=Ts  seed=[23341]
  Clock : Clock
  Constant : Constant  Value=0
  Interval Test for 0s to 200s : simulink/Logic and Bit Operations/Interval Test  IntervalClosedRight=off  uplimit=200  IntervalClosedLeft=on  lowlimit=0  OutDataTypeStr=boolean
  Interval Test for 400s to 600s : simulink/Logic and Bit Operations/Interval Test  IntervalClosedRight=off  uplimit=600  IntervalClosedLeft=off  lowlimit=400  OutDataTypeStr=boolean
  Logical Operator : Logic  Operator=OR  AllPortsSameDT=off  OutDataTypeStr=boolean
  Residual Concentration Reference : Step  Time=tStep  Before=Concentration0  After=2  SampleTime=0
  Sum : Sum  Inputs=|++
  Switch : Switch  Criteria=u2 ~= 0
  Zero-Order Hold : ZeroOrderHold  SampleTime=Ts
  CAref : Outport  VectorParamsAs1DForOutWhenUnconnected=off
  Enable : Outport  Port=2  VectorParamsAs1DForOutWhenUnconnected=off
  wires:
  Constant/1 -> Switch/3
  Band-Limited White Noise/1 -> Switch/1
  Logical Operator/1 -> Zero-Order Hold/1, Switch/2
  Switch/1 -> Sum/1
  Residual Concentration Reference/1 -> Sum/2
  Sum/1 -> CAref/1
  Zero-Order Hold/1 -> Enable/1
  Clock/1 -> Interval Test for 400s to 600s/1, Interval Test for 0s to 200s/1
  Interval Test for 0s to 200s/1 -> Logical Operator/1
  Interval Test for 400s to 600s/1 -> Logical Operator/2

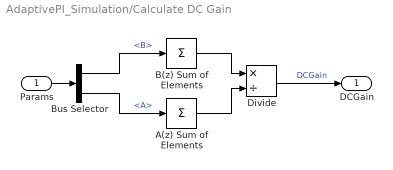
== system AdaptivePI_Simulation/Calculate DC Gain ==
  Params : Inport
  A(z) Sum of Elements : Sum  Inputs=+
  B(z) Sum of Elements : Sum  Inputs=+
  Bus Selector : BusSelector  OutputSignals=B,A
  Divide : Product  Inputs=*/
  DCGain : Outport  VectorParamsAs1DForOutWhenUnconnected=off
  wires:
  A(z) Sum of Elements/1 -> Divide/2
  B(z) Sum of Elements/1 -> Divide/1
  Params/1 -> Bus Selector/1
  Bus Selector/1 -> B(z) Sum of Elements/1  "<B>"
  Bus Selector/2 -> A(z) Sum of Elements/1  "<A>"
  Divide/1 -> DCGain/1  "DCGain"

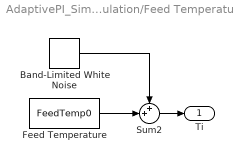
== system AdaptivePI_Simulation/Feed Temperature ==
  Band-Limited White Noise : simulink/Sources/Band-Limited White Noise  Cov=0.0075  Ts=Ts  seed=[23341]
  Feed Temperature : Constant  Value=FeedTemp0
  Sum2 : Sum  Inputs=++|
  Ti : Outport  VectorParamsAs1DForOutWhenUnconnected=off
  wires:
  Band-Limited White Noise/1 -> Sum2/1
  Feed Temperature/1 -> Sum2/2
  Sum2/1 -> Ti/1

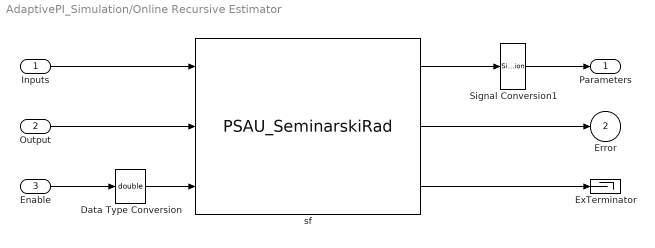
== system AdaptivePI_Simulation/Online Recursive Estimator ==
  Inputs : Inport
  Output : Inport  Port=2
  Enable : Inport  Port=3
  Data Type Conversion : DataTypeConversion  OutDataTypeStr=double
  ExTerminator : Terminator
  Signal Conversion1 : SignalConversion  ConversionOutput=Virtual bus  OverrideOpt=off
  sf : S-Function  InitFcn=try, set_param(gcb,'FunctionName','PSAU_SeminarskiRad'), end  FunctionName=PSAU_SeminarskiRad  Parameters=int32(A0), int32(B0), int32(F0), int32(C0), int32(D0), int32(d), Lambda, P0, int32(ModelStructure), int32(EstimationMethod), int32(WindowLength), Tolerance, SampleTime, int32(History), ProcessNoiseCovariance  SFunctionModules=PSAU_SeminarskiRad_wrapper  SFunctionDeploymentMode=off  EnableBusSupport=off  mask(S-Function Builder){}
      mask help: Simulink:masks:SFunctionBuilder_MD
      mask init:
      | val = [[.9  0.75 0.75 1 1 .9 .9 1]',[1 1 0.75 0.75 .9 .9 1 .9]'];try , sys = get_param(gcb,'SfunBuilderFcnName');if isempty(sys), sys = get_param(gcb,'FunctionName'); end,catch, sys = get_param(gcb,'FunctionName'); end
      settings: CopyFcn=set_param(gcbh,'LinkStatus','none')  PreSaveFcn=try, set_param(gcb,'FunctionName','PSAU_SeminarskiRad'), end  OpenFcn=sfunctionwizard(gcbh)
      mask Display: plot(val(:,1),val(:,2)),disp(sys), port_label('input',1,'u0'), port_label('input',2,'y0'), port_label('input',3,'Enable'), port_label('output',1,'Params'), port_label('output',2,'Error'), port_label('output',3,'Excitation')
  Parameters : Outport
  Error : Outport  Port=2
  wires:
  sf/1 -> Signal Conversion1/1
  Data Type Conversion/1 -> sf/3
  Signal Conversion1/1 -> Parameters/1
  Output/1 -> sf/2
  Inputs/1 -> sf/1
  Enable/1 -> Data Type Conversion/1
  sf/3 -> ExTerminator/1
  sf/2 -> Error/1

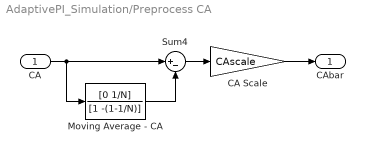
== system AdaptivePI_Simulation/Preprocess CA ==
  CA : Inport
  CA Scale : Gain  Gain=CAscale
  Moving Average - CA : DiscreteFilter  Numerator=[0 1/N]  Denominator=[1 -(1-1/N)]  InitialStates=Concentration0*N  SampleTime=Ts
  Sum4 : Sum  Inputs=|+-
  CAbar : Outport  VectorParamsAs1DForOutWhenUnconnected=off
  wires:
  CA/1 -> Moving Average - CA/1, Sum4/1
  Moving Average - CA/1 -> Sum4/2
  Sum4/1 -> CA Scale/1
  CA Scale/1 -> CAbar/1

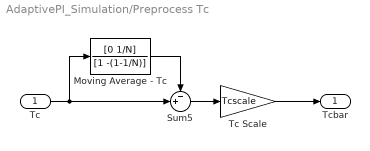
== system AdaptivePI_Simulation/Preprocess Tc ==
  Tc : Inport
  Moving Average - Tc : DiscreteFilter  Numerator=[0 1/N]  Denominator=[1 -(1-1/N)]  InitialStates=CoolantTemp0*N  SampleTime=Ts
  Sum5 : Sum  Inputs=-+|
  Tc Scale : Gain  Gain=Tcscale
  Tcbar : Outport  VectorParamsAs1DForOutWhenUnconnected=off
  wires:
  Tc/1 -> Moving Average - Tc/1, Sum5/2
  Moving Average - Tc/1 -> Sum5/1
  Sum5/1 -> Tc Scale/1
  Tc Scale/1 -> Tcbar/1

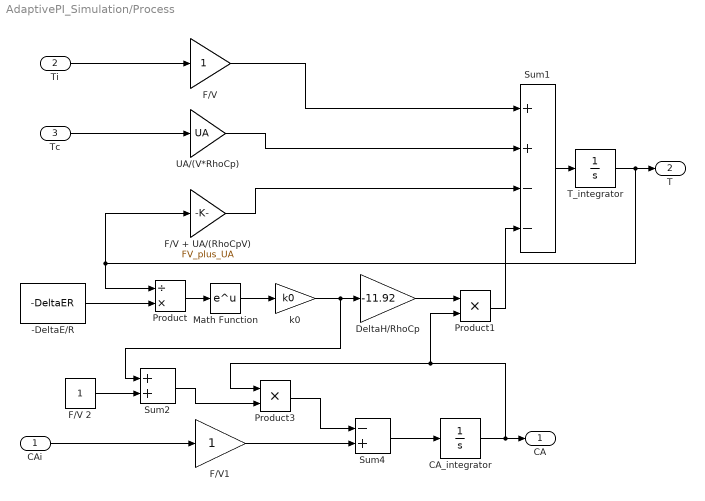
== system AdaptivePI_Simulation/Process ==
  CAi : Inport
  Ti : Inport  Port=2
  Tc : Inport  Port=3
  -DeltaE/R : Constant  Value=-DeltaER
  CA_integrator : Integrator  InitialCondition=Concentration0  LimitOutput=on  LowerSaturationLimit=0
  DeltaH/RhoCp : Gain  Gain=-11.92  SaturateOnIntegerOverflow=on  OutDataTypeStr=Inherit: Same as input  ParamDataTypeStr=Inherit: Same as input
  F/V : Gain  SaturateOnIntegerOverflow=on  OutDataTypeStr=Inherit: Same as input  ParamDataTypeStr=Inherit: Same as input
  F/V + UA/(RhoCpV) : Gain  Gain=FV_plus_UA  SaturateOnIntegerOverflow=on  OutDataTypeStr=Inherit: Same as input  ParamDataTypeStr=Inherit: Same as input
  F/V 2 : Constant
  F/V1 : Gain  SaturateOnIntegerOverflow=on  OutDataTypeStr=Inherit: Same as input  ParamDataTypeStr=Inherit: Same as input
  Math Function : Math  SignedPower=on  SaturateOnIntegerOverflow=on
  Product : Product  Inputs=/*  InputSameDT=on  RndMeth=Zero  SaturateOnIntegerOverflow=on  OutDataTypeStr=Inherit: Same as first input
  Product1 : Product  InputSameDT=on  RndMeth=Zero  SaturateOnIntegerOverflow=on  OutDataTypeStr=Inherit: Same as first input
  Product3 : Product  InputSameDT=on  RndMeth=Zero  SaturateOnIntegerOverflow=on  OutDataTypeStr=Inherit: Same as first input
  Sum1 : Sum  Inputs=++--  InputSameDT=on  SaturateOnIntegerOverflow=on  OutDataTypeStr=Inherit: Same as first input
  Sum2 : Sum  InputSameDT=on  SaturateOnIntegerOverflow=on  OutDataTypeStr=Inherit: Same as first input
  Sum4 : Sum  Inputs=-+  InputSameDT=on  SaturateOnIntegerOverflow=on  OutDataTypeStr=Inherit: Same as first input
  T_integrator : Integrator  InitialCondition=ReactorTemp0  LimitOutput=on  LowerSaturationLimit=0
  UA/(V*RhoCp) : Gain  Gain=UA  SaturateOnIntegerOverflow=on  OutDataTypeStr=Inherit: Same as input  ParamDataTypeStr=Inherit: Same as input
  k0 : Gain  Gain=k0  SaturateOnIntegerOverflow=on  OutDataTypeStr=Inherit: Same as input  ParamDataTypeStr=Inherit: Same as input
  CA : Outport  VectorParamsAs1DForOutWhenUnconnected=off
  T : Outport  Port=2  VectorParamsAs1DForOutWhenUnconnected=off
  wires:
  F/V/1 -> Sum1/1
  Sum1/1 -> T_integrator/1
  T_integrator/1 -> Product/1, F/V + UA/(RhoCpV)/1, T/1
  UA/(V*RhoCp)/1 -> Sum1/2
  F/V + UA/(RhoCpV)/1 -> Sum1/3
  Product/1 -> Math Function/1
  Math Function/1 -> k0/1
  DeltaH/RhoCp/1 -> Product1/1
  Product1/1 -> Sum1/4
  k0/1 -> DeltaH/RhoCp/1, Sum2/1
  -DeltaE/R/1 -> Product/2
  Product3/1 -> Sum4/1
  Sum4/1 -> CA_integrator/1
  CA_integrator/1 -> Product1/2, Product3/1, CA/1
  F/V 2/1 -> Sum2/2
  F/V1/1 -> Sum4/2
  Ti/1 -> F/V/1
  CAi/1 -> F/V1/1
  Tc/1 -> UA/(V*RhoCp)/1
  Sum2/1 -> Product3/2

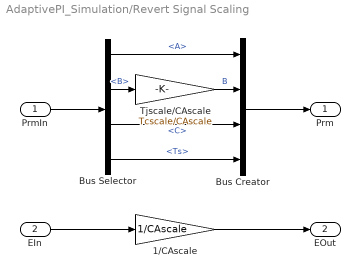
== system AdaptivePI_Simulation/Revert Signal Scaling ==
  PrmIn : Inport
  EIn : Inport  Port=2
  1/CAscale : Gain  Gain=1/CAscale
  Bus Creator : BusCreator  Inputs=4
  Bus Selector : BusSelector  OutputSignals=A,B,C,Ts
  Tjscale/CAscale : Gain  Gain=Tcscale/CAscale
  Prm : Outport  VectorParamsAs1DForOutWhenUnconnected=off
  EOut : Outport  Port=2  VectorParamsAs1DForOutWhenUnconnected=off
  wires:
  EIn/1 -> 1/CAscale/1
  PrmIn/1 -> Bus Selector/1
  Bus Selector/1 -> Bus Creator/1  "<A>"
  Bus Selector/4 -> Bus Creator/4  "<Ts>"
  Bus Selector/3 -> Bus Creator/3  "<C>"
  Bus Selector/2 -> Tjscale/CAscale/1  "<B>"
  Tjscale/CAscale/1 -> Bus Creator/2  "B"
  1/CAscale/1 -> EOut/1
  Bus Creator/1 -> Prm/1

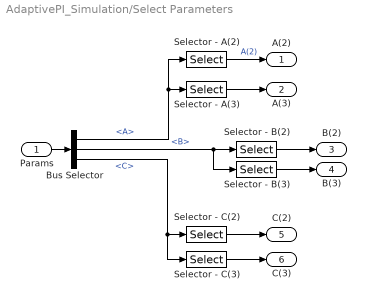
== system AdaptivePI_Simulation/Select Parameters ==
  Params : Inport
  Bus Selector : BusSelector  OutputSignals=A,B,C
  Selector - A(2) : Selector  NumberOfDimensions=2  InputPortWidth=3  IndexOptions=Index vector (dialog),Index vector (dialog)  Indices=1,2  OutputSizes=1,1
  Selector - A(3) : Selector  NumberOfDimensions=2  InputPortWidth=3  IndexOptions=Index vector (dialog),Index vector (dialog)  Indices=1,3  OutputSizes=1,1
  Selector - B(2) : Selector  NumberOfDimensions=2  InputPortWidth=3  IndexOptions=Index vector (dialog),Index vector (dialog)  Indices=1,2  OutputSizes=1,1
  Selector - B(3) : Selector  NumberOfDimensions=2  InputPortWidth=3  IndexOptions=Index vector (dialog),Index vector (dialog)  Indices=1,3  OutputSizes=1,1
  Selector - C(2) : Selector  NumberOfDimensions=2  InputPortWidth=3  IndexOptions=Index vector (dialog),Index vector (dialog)  Indices=1,2  OutputSizes=1,1
  Selector - C(3) : Selector  NumberOfDimensions=2  InputPortWidth=3  IndexOptions=Index vector (dialog),Index vector (dialog)  Indices=1,3  OutputSizes=1,1
  A(2) : Outport  VectorParamsAs1DForOutWhenUnconnected=off
  A(3) : Outport  Port=2  VectorParamsAs1DForOutWhenUnconnected=off
  B(2) : Outport  Port=3  VectorParamsAs1DForOutWhenUnconnected=off
  B(3) : Outport  Port=4  VectorParamsAs1DForOutWhenUnconnected=off
  C(2) : Outport  Port=5  VectorParamsAs1DForOutWhenUnconnected=off
  C(3) : Outport  Port=6  VectorParamsAs1DForOutWhenUnconnected=off
  wires:
  Params/1 -> Bus Selector/1
  Bus Selector/1 -> Selector - A(2)/1, Selector - A(3)/1  "<A>"
  Bus Selector/2 -> Selector - B(3)/1, Selector - B(2)/1  "<B>"
  Bus Selector/3 -> Selector - C(3)/1, Selector - C(2)/1  "<C>"
  Selector - A(3)/1 -> A(3)/1
  Selector - A(2)/1 -> A(2)/1  "A(2)"
  Selector - B(2)/1 -> B(2)/1
  Selector - B(3)/1 -> B(3)/1
  Selector - C(2)/1 -> C(2)/1
  Selector - C(3)/1 -> C(3)/1

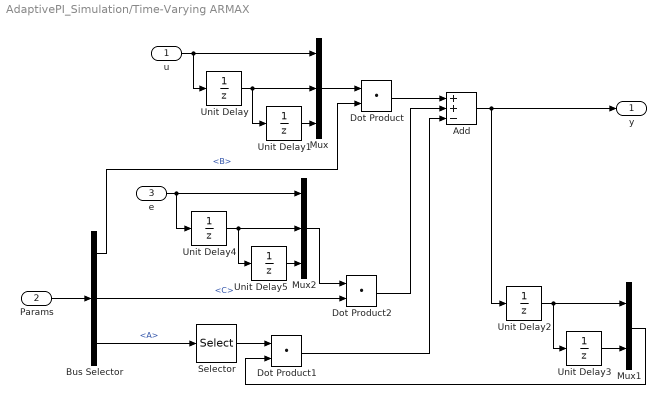
== system AdaptivePI_Simulation/Time-Varying ARMAX ==
  u : Inport
  Params : Inport  Port=2
  e : Inport  Port=3
  Add : Sum  Inputs=++-
  Bus Selector : BusSelector  OutputSignals=B,C,A
  Dot Product : DotProduct  InputSameDT=on  OutDataTypeStr=Inherit: Inherit via internal rule
  Dot Product1 : DotProduct  InputSameDT=on  OutDataTypeStr=Inherit: Inherit via internal rule
  Dot Product2 : DotProduct  InputSameDT=on  OutDataTypeStr=Inherit: Inherit via internal rule
  Mux : Mux  Inputs=3
  Mux1 : Mux  Inputs=2
  Mux2 : Mux  Inputs=3
  Selector : Selector  NumberOfDimensions=2  InputPortWidth=3  IndexOptions=Index vector (dialog),Index vector (dialog)  Indices=1,[2 3]  OutputSizes=1,1
  Unit Delay{,1..5} (6 alike) : UnitDelay  SampleTime=-1  HasFrameUpgradeWarning=on
  y : Outport  VectorParamsAs1DForOutWhenUnconnected=off
  wires:
  Unit Delay/1 -> Unit Delay1/1, Mux/2
  Mux/1 -> Dot Product/1
  Bus Selector/1 -> Dot Product/2  "<B>"
  Unit Delay1/1 -> Mux/3
  u/1 -> Unit Delay/1, Mux/1
  Bus Selector/3 -> Selector/1  "<A>"
  Add/1 -> y/1, Unit Delay2/1
  Unit Delay2/1 -> Unit Delay3/1, Mux1/1
  Dot Product/1 -> Add/1
  Unit Delay3/1 -> Mux1/2
  Selector/1 -> Dot Product1/1
  e/1 -> Unit Delay4/1, Mux2/1
  Bus Selector/2 -> Dot Product2/2  "<C>"
  Dot Product1/1 -> Add/3
  Mux1/1 -> Dot Product1/2
  Dot Product2/1 -> Add/2
  Params/1 -> Bus Selector/1
  Unit Delay4/1 -> Unit Delay5/1, Mux2/2
  Unit Delay5/1 -> Mux2/3
  Mux2/1 -> Dot Product2/1
